simulink model "sampleModel2"  (Simulink 8.9)
settings: Solver=VariableStepAuto  StartTime=0.0  StopTime=10.0  RelTol=1e-3
undefined symbols (not defined in the file): DiscIntNeverNeededParam
libraries: simulink x1
settings Model: SuppressorTable=22 serialization::archive 11 0 6 0 0 0 11 0  Creator=cyfuzz  LastModifiedBy=cyfuzz
settings DataIOCC: LimitDataPoints=off  SaveFormat=Dataset  SignalLoggingSaveFormat=Dataset
settings OptimizationCC: LifeSpan=auto
settings DebuggingCC: UnderspecifiedInitializationDetection=Simplified  MergeDetectMultiDrivingBlocksExec=error  FcnCallInpInsideContextMsg=error  StateNameClashWarn=none  SFUnexpectedBacktrackingDiag=error  SFNoUnconditionalDefaultTransitionDiag=error  SFExecutionAtInitializationDiag=warning
settings HardwareCC: ProdBitPerPointer=64  ProdBitPerSizeT=64  ProdBitPerPtrDiffT=64  ProdLargestAtomicFloat=Float  ProdIntDivRoundTo=Zero  ProdEndianess=LittleEndian  ProdWordSize=64  ProdHWDeviceType=Intel->x86-64 (Windows64)
settings ModelReferenceCC: PropagateSignalLabelsOutOfModel=on
settings GRTTargetCC: TargetLangStandard=C99 (ISO)  GeneratePreprocessorConditionals=Use local settings  CombineOutputUpdateFcns=on  GRTInterface=off
settings ConfigComp: CovMetricSettings=dwe  CovHtmlReporting=off  CovSaveCumulativeToWorkspaceVar=off  CovSaveSingleToWorkspaceVar=off  CovExternalEMLEnable=on

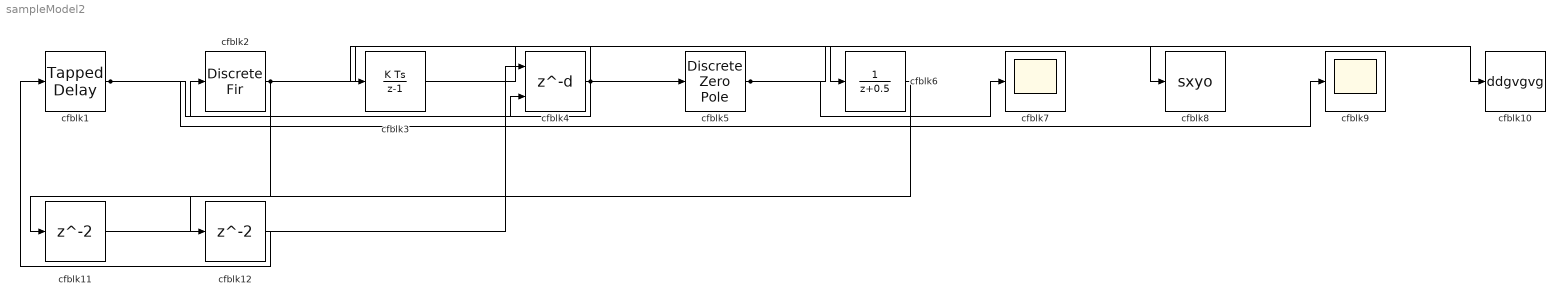
== system sampleModel2 ==
  cfblk1 : simulink/Discrete/Tapped Delay  vinit=0.0  samptime=-1  NumDelays=1  DelayOrder=Oldest  includeCurrent=off
  cfblk10 : ToWorkspace  VariableName=ddgvgvg  SaveFormat=Timeseries  SampleTime=-1
  cfblk11 : Delay  SampleTime=1
  cfblk12 : Delay  SampleTime=1
  cfblk2 : DiscreteFir  SampleTime=1
  cfblk3 : DiscreteIntegrator  InitialConditionSetting=State (most efficient)  ICPrevOutput=DiscIntNeverNeededParam  ICPrevScaledInput=DiscIntNeverNeededParam
  cfblk4 : Delay  DelayLengthSource=Input port  SampleTime=1
      settings: InputPortMap=u0,p1
  cfblk5 : DiscreteZeroPole  Poles=[0 0.5]  Gain=1
  cfblk6 : DiscreteTransferFcn  SampleTime=1
  cfblk7 : Scope
  cfblk8 : ToFile  Filename=sxyo  SaveFormat=Timeseries
  cfblk9 : Scope
  wires:
  cfblk3/1 -> cfblk10/1
  cfblk4/1 -> cfblk2/1, cfblk5/1, cfblk3/1
  cfblk2/1 -> cfblk6/1, cfblk12/1
  cfblk5/1 -> cfblk7/1, cfblk8/1
  cfblk1/1 -> cfblk9/1, cfblk4/2
  cfblk6/1 -> cfblk11/1
  cfblk11/1 -> cfblk4/1
  cfblk12/1 -> cfblk1/1
